simulink model "Observador"  (R2022b)
settings: Solver=VariableStepAuto  StartTime=0.0  StopTime=10.0  RelTol=1e-3
values from neighbouring files (symbols this model uses):
  A = [-1 -2 ... (first row only)    [ABinvariantes11deJunio.m]    (also in Convertibility.m = [0 1 0  0 0; DivirsoresElementales.m = [1 0 -1; 0 1 0; 0 0 2]; Examen.m = [1 1;0 1]; Examen2.m = [0 0  0 0 0)
  B = [1 ... (first row only)    [ABinvariantes11deJunio.m]    (also in Convertibility.m = [0 0; Examen.m = [1;0]; Examen2.m = [1 0; Sestrella.m = [0;1;0])
  C = [1 0]    [Examen.m]    (also in Sestrella.m = [0 1 0; 0 0 1]; Westrella.m = [0 1 0; 0 0 1])
  F = place(A,B,P)    [Examen2.m]    (also in Westrella.m = P*A0*Pr)
  G = P*B    [Westrella.m]
  L = [0 ;0; 1]    [Sestrella.m]    (also in Westrella.m)
  M = C*Pr    [Westrella.m]
settings Model: Creator=raul  LastModifiedBy=raul

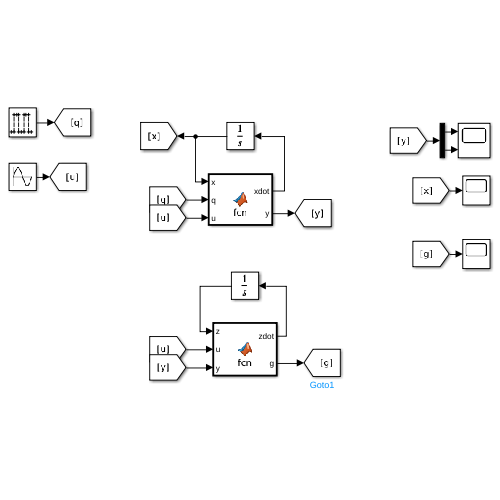
[thumbnail: Simulink's stored preview of the top-level diagram]
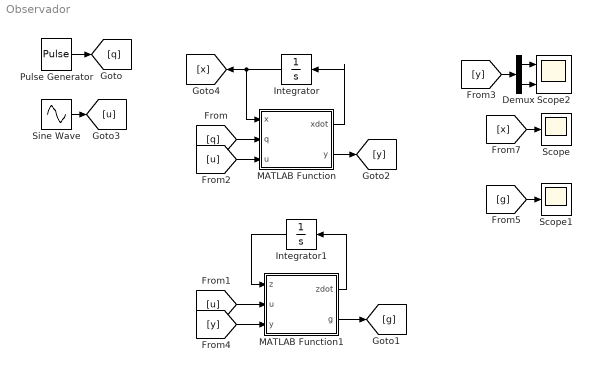
== system Observador ==
  Demux : Demux  Outputs=2
  Integrator : Integrator  InitialCondition=[0;0;0]
  Integrator1 : Integrator  InitialCondition=[0;0]
  MATLAB Function : MATLAB Function  TreatAsAtomicUnit=on
  MATLAB Function1 : MATLAB Function  TreatAsAtomicUnit=on
  Pulse Generator : DiscretePulseGenerator  Period=10  PulseWidth=5
  Scope : Scope
  Scope1 : Scope
  Scope2 : Scope  NumInputPorts=2
  Sine Wave : Sin  SampleTime=0
  wires:
  Pulse Generator/1 -> [q]
  MATLAB Function/1(xdot) -> Integrator/1
  MATLAB Function/2(y) -> [y]
  [q] -> MATLAB Function/2(q)
  [u] -> MATLAB Function/3(u)
  Integrator/1 -> [x], MATLAB Function/1(x)
  MATLAB Function1/1(zdot) -> Integrator1/1
  Integrator1/1 -> MATLAB Function1/1(z)
  [u] -> MATLAB Function1/2(u)
  [y] -> MATLAB Function1/3(y)
  MATLAB Function1/2(g) -> [g]
  [g] -> Scope1/1
  [x] -> Scope/1
  Sine Wave/1 -> [u]
  Demux/1 -> Scope2/1
  Demux/2 -> Scope2/2
  [y] -> Demux/1

== matlab function Observador/MATLAB Function1 ==
  data: zdot output; z input; u input; y input; g output; F parameter; M parameter; G parameter; E parameter
function [zdot,g] = fcn(z,u,y,F, M, G, E)

zdot=F*z+G*u-E*y;
g=M*z;

== matlab function Observador/MATLAB Function ==
  data: x input; xdot output; q input; u input; y output; A parameter; B parameter; C parameter; L parameter
function [xdot,y] = fcn(x,q,u,A, B, C, L)

xdot=A*x+B*u+L*q;
y=C*x;
